simulink model "Car"  (R2023a)
settings: Solver=ode45  StartTime=0.0  StopTime=PROFILE_LENGTH  MaxStep=300.0  RelTol=1e-3
values from neighbouring files (symbols this model uses):
  AIR_DENSITY = 1.2    [Setup.m]
  C_ROLLING_RESISTANCE = .0025    (= 0.0025)    [Setup.m]
  DRAG_COEFFICIENT = 0.25    [Setup.m]
  DRIVER_DISPLAY_DRAW = 2.5    [Setup.m]
  FAN_DRAW = 4.8    [Setup.m]
  FRONTAL_AREA = 1    [Setup.m]    (also in init.m = 1.262)
  FULL_PACK_KWH = HV_PACK_VOLTAGE * HV_PACK_CAPACITY * UNIT_TO_KILO    (= 7.68)    [Setup.m]    (also in init.m)
  GRAVITY = 9.81    [Setup.m]
  HEADLIGHT_DRAW = 2    [Setup.m]
  HV_PACK_VOLTAGE = 96    [Setup.m]    (also in init.m)
  INT_CURRENTS = CURRENT_DATA_ECO(1):0.0001:CURRENT_DATA_ECO(end)    [Setup.m]
  INT_DISTANCES = DISTANCE(1):0.25:DISTANCE(end)    [Setup.m]
  INT_GRADE_ANGLE = interp1(DISTANCE, GRADE_ANGLE, INT_DISTANCES,'spline')    [Setup.m]
  INT_TORQUES_ECO = interp1(CURRENT_DATA_ECO, TORQUES_DATA_ECO, INT_CURRENTS,'spline')    [Setup.m]
  MAX_CURRENT = max(CURRENT_DATA_ECO)    [Setup.m]
  MAX_TORQUE = max(TORQUES_DATA_ECO)    [Setup.m]
  SECONDS_PER_HOUR = 3600    [Setup.m]    (also in init.m)
  START_TIME = 9*(SECONDS_PER_HOUR) + 0*(SECONDS_PER_MINUTE)    (= 32400)    [Setup.m]    (also in init.m = 0)
  STARTING_KWH = FULL_PACK_KWH * (1 - 0)    (= 7.68)    [Setup.m]    (also in init.m)
  TARGET_SPEED = 10    [Setup.m]
  TOTAL_MASS = CAR_MASS + DRIVER_MASS    (= 282.996279643)    [Setup.m]    (also in init.m)
  UNIT_TO_KILO = 1 / 1000    (= 0.001)    [Setup.m]    (also in init.m)
  WHEEL_RADIUS = WHEEL_DIAMETER_METERS / 2    (= 0.2794)    [Setup.m]
libraries: slpidlib x1
settings Model: Creator=jcpetrie  LastModifiedBy=gluo25
settings SolverCC: ZeroCrossAlgorithm=Adaptive
settings ModelReferenceCC: EnableRefExpFcnMdlSchedulingChecks=on

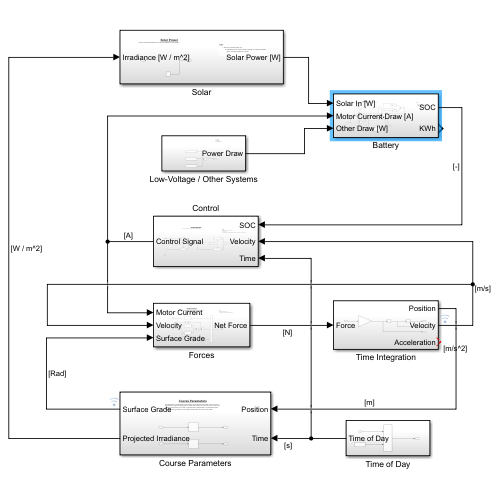
[thumbnail: Simulink's stored preview of the top-level diagram]
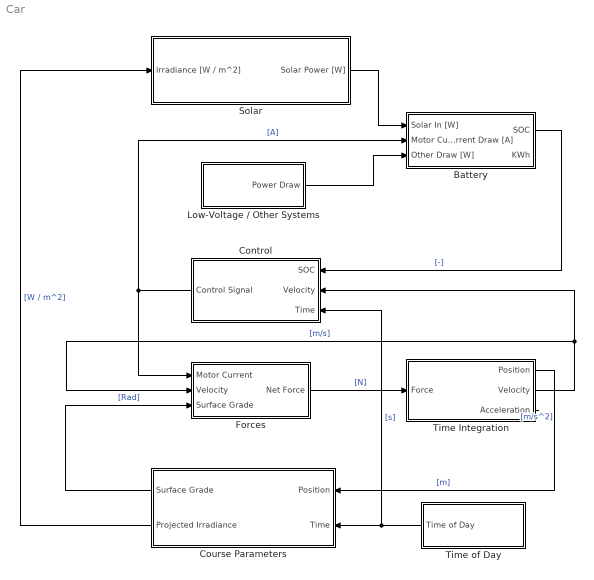
== system Car ==
  Battery : Subsystem
  Control : Subsystem
  Course Parameters : Subsystem
  Forces : Subsystem
  Low-Voltage / Other Systems : Subsystem
  Solar : Subsystem
  Time Integration : Subsystem
  Time of Day : Subsystem
  wires:
  Control/1(Control Signal) -> Battery/2(Motor Current Draw [A]), Forces/1(Motor Current)  "[A]"
  Time Integration/2(Velocity) -> Forces/2(Velocity), Control/2(Velocity)  "[m/s]"
  Forces/1(Net Force) -> Time Integration/1(Force)  "[N]"
  Time Integration/1(Position) -> Course Parameters/1(Position)  "[m]"
  Time Integration/3(Acceleration) -> ?  "[m/s^2]"
  Battery/1(SOC) -> Control/1(SOC)  "[-]"
  Course Parameters/1(Surface Grade) -> Forces/3(Surface Grade)  "[Rad]"
  Time of Day/1(Time of Day) -> Control/3(Time), Course Parameters/2(Time)  "[s]"
  Low-Voltage / Other Systems/1(Power Draw) -> Battery/3(Other Draw [W])
  Solar/1(Solar Power [W]) -> Battery/1(Solar In [W])
  Course Parameters/2(Projected Irradiance) -> Solar/1(Irradiance [W / m^2])  "[W / m^2]"

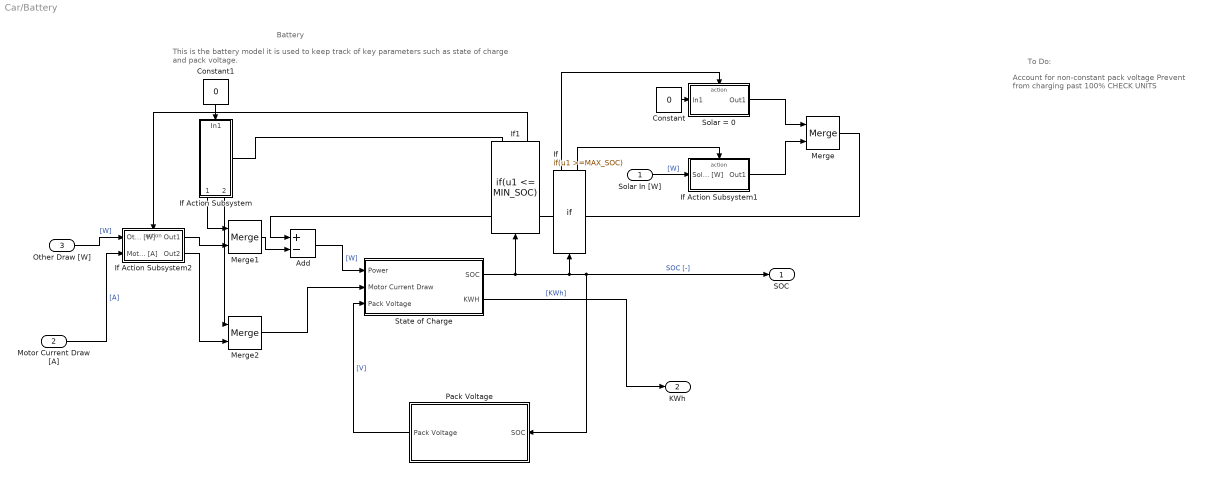
== system Car/Battery ==
  note: To Do:
  note: Battery
  note: This is the battery model it is used to keep track of key parameters such as state of charge and pack voltage.
  note: Account for non-constant pack voltage
      | Prevent from charging past 100%
      | CHECK UNITS
  Solar In [W] : Inport
  Motor Current Draw [A] : Inport  Port=2
  Other Draw [W] : Inport  Port=3
  Add : Sum  Inputs=+-
  Constant : Constant  Value=0
  Constant1 : Constant  Value=0
  If : If  IfExpression=u1 >=MAX_SOC  ZeroCross=off
  If Action Subsystem : Subsystem  TreatAsAtomicUnit=on
  If Action Subsystem1 : Subsystem  TreatAsAtomicUnit=on
  If Action Subsystem2 : Subsystem  TreatAsAtomicUnit=on
  If1 : If  IfExpression=u1 <= MIN_SOC  ZeroCross=off
  Merge : Merge
  Merge1 : Merge
  Merge2 : Merge
  Pack Voltage : Subsystem
  Solar = 0 : Subsystem  TreatAsAtomicUnit=on
  State of Charge : Subsystem
  SOC : Outport
  KWh : Outport  Port=2
  wires:
  Motor Current Draw [A]/1 -> If Action Subsystem2/2(Motor Current Draw [A])  "[A]"
  State of Charge/1(SOC) -> SOC/1, Pack Voltage/1(SOC), If/1, If1/1  "SOC [-]"
  Pack Voltage/1(Pack Voltage) -> State of Charge/3(Pack Voltage)  "[V]"
  State of Charge/2(KWH) -> KWh/1  "[KWh]"
  Solar In [W]/1 -> If Action Subsystem1/1(Solar In [W])  "[W]"
  Add/1 -> State of Charge/1("Power ")  "[W]"
  If/1 -> Solar = 0/Action
  Constant/1 -> Solar = 0/1(In1)
  If/2 -> If Action Subsystem1/Action
  Solar = 0/1(Out1) -> Merge/1
  Merge/1 -> Add/1
  Other Draw [W]/1 -> If Action Subsystem2/1(Other Draw [W])  "[W]"
  If Action Subsystem1/1(Out1) -> Merge/2
  If1/1 -> If Action Subsystem/Action
  Constant1/1 -> If Action Subsystem/1(In1)
  If1/2 -> If Action Subsystem2/Action
  If Action Subsystem2/1(Out1) -> Merge1/2
  If Action Subsystem/1(Out1) -> Merge1/1
  Merge1/1 -> Add/2
  Merge2/1 -> State of Charge/2(Motor Current Draw)
  If Action Subsystem2/2(Out2) -> Merge2/2
  If Action Subsystem/2(Out2) -> Merge2/1

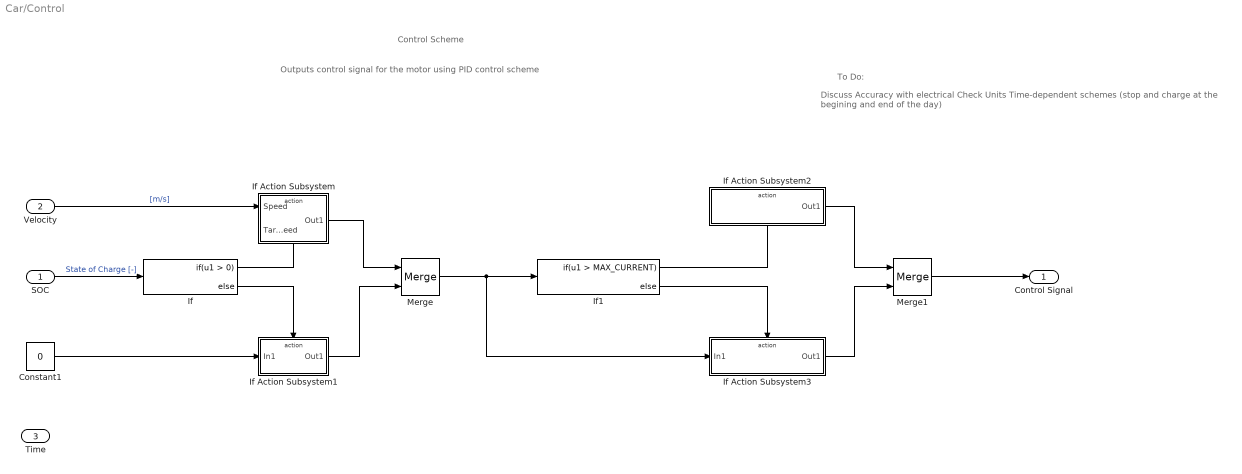
== system Car/Control ==
  note: Outputs control signal for the motor using PID control scheme
  note: To Do:
  note: Control Scheme
  note: Discuss Accuracy with electrical
      | Check Units
      | Time-dependent schemes (stop and charge at the begining and end of the day)
  SOC : Inport
  Velocity : Inport  Port=2
  Time : Inport  Port=3
  Constant1 : Constant  Value=0
  If : If  ZeroCross=off
  If Action Subsystem : Subsystem  TreatAsAtomicUnit=on
  If Action Subsystem1 : Subsystem  TreatAsAtomicUnit=on
  If Action Subsystem2 : Subsystem  TreatAsAtomicUnit=on
  If Action Subsystem3 : Subsystem  TreatAsAtomicUnit=on
  If1 : If  IfExpression=u1 > MAX_CURRENT
  Merge : Merge
  Merge1 : Merge
  Control Signal : Outport
  wires:
  Velocity/1 -> If Action Subsystem/1(Speed)  "[m/s]"
  SOC/1 -> If/1  "State of Charge [-]"
  If/1 -> If Action Subsystem/Action
  If/2 -> If Action Subsystem1/Action
  Constant1/1 -> If Action Subsystem1/1(In1)
  If Action Subsystem/1(Out1) -> Merge/1
  If Action Subsystem1/1(Out1) -> Merge/2
  Merge/1 -> If Action Subsystem3/1(In1), If1/1
  If1/1 -> If Action Subsystem2/Action
  Merge1/1 -> Control Signal/1
  If Action Subsystem2/1(Out1) -> Merge1/1
  If1/2 -> If Action Subsystem3/Action
  If Action Subsystem3/1(Out1) -> Merge1/2

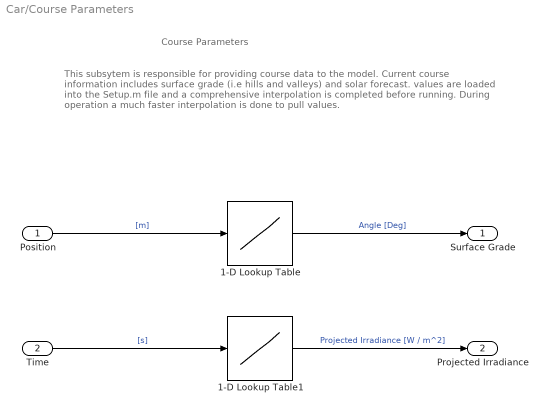
== system Car/Course Parameters ==
  note: Course Parameters
  note: This subsytem is responsible for providing course data to the model. Current course information includes surface grade (i.e hills and valleys) and solar forecast. values are loaded into the Setup.m file and a comprehensive interpolation is completed before running. During operation a much faster interpolation is done to pull values.
  Position : Inport
  Time : Inport  Port=2
  1-D Lookup Table : Lookup_n-D  NumberOfTableDimensions=1  BreakpointsForDimension1=INT_DISTANCES  Table=INT_GRADE_ANGLE  InternalRulePriority=Speed  RndMeth=Simplest
  1-D Lookup Table1 : Lookup_n-D  NumberOfTableDimensions=1  BreakpointsForDimension1=[-5:5]  Table=tanh([-5:5])  InternalRulePriority=Speed  RndMeth=Simplest
  Surface Grade : Outport
  Projected Irradiance : Outport  Port=2
  wires:
  Position/1 -> 1-D Lookup Table/1  "[m]"
  Time/1 -> 1-D Lookup Table1/1  "[s]"
  1-D Lookup Table/1 -> Surface Grade/1  "Angle [Deg]"
  1-D Lookup Table1/1 -> Projected Irradiance/1  "Projected Irradiance [W / m^2]"

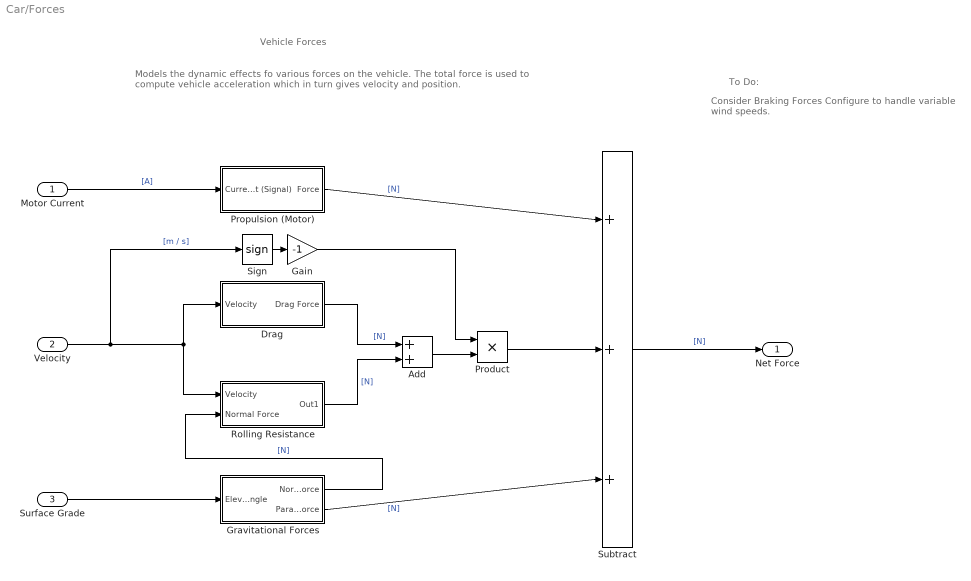
== system Car/Forces ==
  note: To Do:
  note: Vehicle Forces
  note: Models the dynamic effects fo various forces on the vehicle. The total force is used to compute vehicle acceleration which in turn gives velocity and position.
  note: Consider Braking Forces
      | Configure to handle variable wind speeds.
  Motor Current : Inport
  Velocity : Inport  Port=2
  Surface Grade : Inport  Port=3
  Add : Sum
  Drag : Subsystem
  Gain : Gain  Gain=-1
  Gravitational Forces : Subsystem
  Product : Product
  Propulsion (Motor) : Subsystem
  Rolling Resistance : Subsystem
  Sign : Signum
  Subtract : Sum  Inputs=+|+|+
  Net Force : Outport
  wires:
  Velocity/1 -> Sign/1, Drag/1(Velocity), Rolling Resistance/1(Velocity)  "[m / s]"
  Propulsion (Motor)/1(Force) -> Subtract/1  "[N]"
  Drag/1(Drag Force) -> Add/1  "[N]"
  Rolling Resistance/1(Out1) -> Add/2  "[N]"
  Subtract/1 -> Net Force/1  "[N]"
  Motor Current/1 -> Propulsion (Motor)/1(Current (Signal))  "[A]"
  Surface Grade/1 -> Gravitational Forces/1(Elevation Angle)
  Gravitational Forces/2(Parallel Force) -> Subtract/3  "[N]"
  Gravitational Forces/1(Normal Force) -> Rolling Resistance/2(Normal Force)  "[N]"
  Sign/1 -> Gain/1
  Add/1 -> Product/2
  Gain/1 -> Product/1
  Product/1 -> Subtract/2

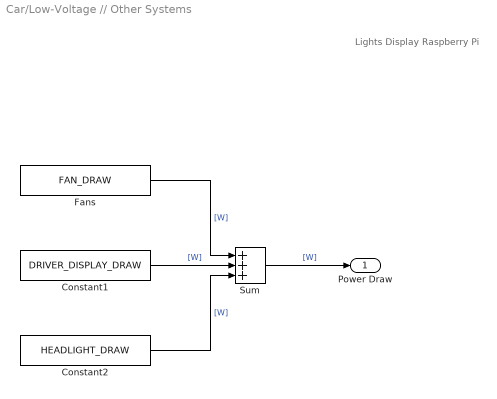
== system Car/Low-Voltage // Other Systems ==
  note: Lights
      | Display
      | Raspberry Pi
  Constant1 : Constant  Value=DRIVER_DISPLAY_DRAW
  Constant2 : Constant  Value=HEADLIGHT_DRAW
  Fans : Constant  Value=FAN_DRAW
  Sum : Sum  Inputs=+++
  Power Draw : Outport
  wires:
  Constant1/1 -> Sum/2  "[W]"
  Sum/1 -> Power Draw/1  "[W]"
  Fans/1 -> Sum/1  "[W]"
  Constant2/1 -> Sum/3  "[W]"

== system Car/Solar ==
  note: Remove constant power out
      | Replace with conversion function based on experimental data which converts irradiance to power
  note: Converts expected irradiance to solar out. Based on testing data.
  note: Solar Power
  note: To Do:
  Irradiance [W / m^2] : Inport
  Constant : Constant  Value=100
  Solar Power [W] : Outport
  wires:
  Constant/1 -> Solar Power [W]/1  "[W]"

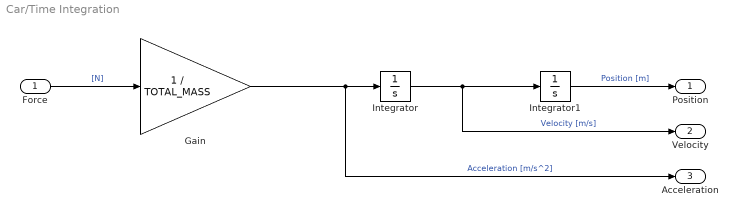
== system Car/Time Integration ==
  Force : Inport
  Gain : Gain  Gain=1 / TOTAL_MASS
  Integrator : Integrator
  Integrator1 : Integrator
  Position : Outport
  Velocity : Outport  Port=2
  Acceleration : Outport  Port=3
  wires:
  Gain/1 -> Acceleration/1, Integrator/1  "Acceleration [m/s^2]"
  Integrator/1 -> Velocity/1, Integrator1/1  "Velocity [m/s]"
  Force/1 -> Gain/1  "[N]"
  Integrator1/1 -> Position/1  "Position [m]"

== system Car/Time of Day ==
  Add : Sum
  Clock : Clock
  Constant : Constant  Value=START_TIME
  Time of Day : Outport
  wires:
  Add/1 -> Time of Day/1  "Time of Day [s]"
  Clock/1 -> Add/1  "Simulation Time [s]"
  Constant/1 -> Add/2  "Start time of day [s]"

== system Car/Battery/If Action Subsystem ==
  In1 : Inport
  Action Port : ActionPort  ActionPortLabel=if(u1 <= MIN_SOC)
  Out1 : Outport
  Out2 : Outport  Port=2
  wires:
  In1/1 -> Out2/1, Out1/1

== system Car/Battery/If Action Subsystem1 ==
  Solar In [W] : Inport
  Action Port : ActionPort  ActionPortLabel=else
  Out1 : Outport
  wires:
  Solar In [W]/1 -> Out1/1

== system Car/Battery/If Action Subsystem2 ==
  Other Draw [W] : Inport
  Motor Current Draw [A] : Inport  Port=2
  Action Port : ActionPort  ActionPortLabel=else
  Out1 : Outport
  Out2 : Outport  Port=2
  wires:
  Other Draw [W]/1 -> Out1/1
  Motor Current Draw [A]/1 -> Out2/1

== system Car/Battery/Pack Voltage ==
  note: Battery Voltage
  note: Outputs the Voltage of the battery given the state of charge
  note: To Do:
  note: Get voltage curve from battery, implment non constant behavior.
  SOC : Inport
  Constant : Constant  Value=HV_PACK_VOLTAGE
  Pack Voltage : Outport
  wires:
  SOC/1 -> ?
  Constant/1 -> Pack Voltage/1  "[V]"

== system Car/Battery/Solar = 0 ==
  In1 : Inport
  Action Port : ActionPort  ActionPortLabel=if(u1 >=MAX_SOC)
  Out1 : Outport
  wires:
  In1/1 -> Out1/1

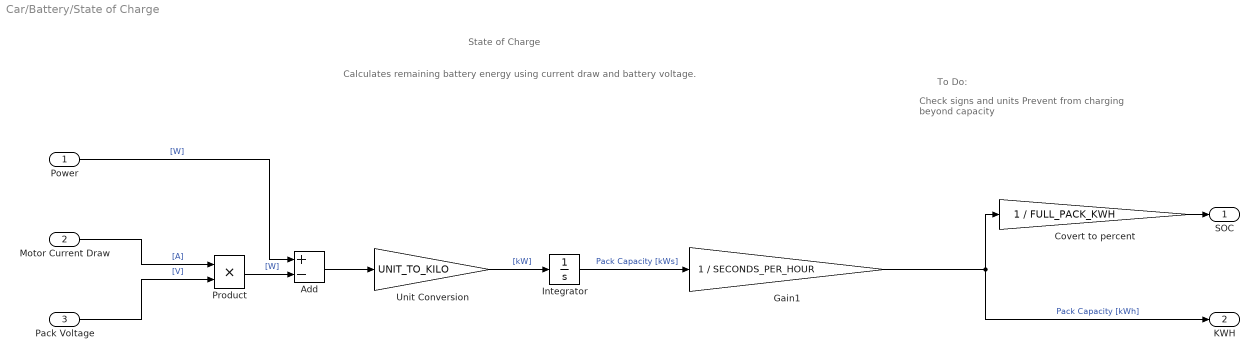
== system Car/Battery/State of Charge ==
  note: State of Charge
  note: Check signs and units
      | Prevent from charging beyond capacity
  note: To Do:
  note: Calculates remaining battery energy using current draw and battery voltage.
  "Power " : Inport
  Motor Current Draw : Inport  Port=2
  Pack Voltage : Inport  Port=3
  Add : Sum  Inputs=+-
  Covert to percent : Gain  Gain=1 / FULL_PACK_KWH
  Gain1 : Gain  Gain=1 / SECONDS_PER_HOUR
  Integrator : Integrator  InitialCondition=STARTING_KWH * SECONDS_PER_HOUR
  Product : Product  Inputs=**
  Unit Conversion : Gain  Gain=UNIT_TO_KILO
  SOC : Outport
  KWH : Outport  Port=2
  wires:
  Integrator/1 -> Gain1/1  "Pack Capacity [kWs]"
  Covert to percent/1 -> SOC/1
  Pack Voltage/1 -> Product/2  "[V]"
  Product/1 -> Add/2  "[W]"
  Unit Conversion/1 -> Integrator/1  "[kW]"
  Motor Current Draw/1 -> Product/1  "[A]"
  Gain1/1 -> KWH/1, Covert to percent/1  "Pack Capacity [kWh]"
  "Power "/1 -> Add/1  "[W]"
  Add/1 -> Unit Conversion/1

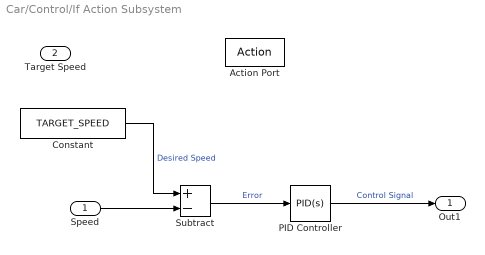
== system Car/Control/If Action Subsystem ==
  Speed : Inport
  Target Speed : Inport  Port=2
  Action Port : ActionPort  ActionPortLabel=if(u1 > 0)
  Constant : Constant  Value=TARGET_SPEED
  PID Controller : slpidlib/PID Controller  Controller=PID  Form=Parallel  TimeDomain=Continuous-time  UseExternalTs=off  SampleTime=-1  IntegratorMethod=Forward Euler  FilterMethod=Forward Euler  ControllerParametersSource=internal  P=2.5  I=0.1  UseKiTs=off  D=0  N=100  UseFilter=on  TunerSelectOption=Transfer Function Based (PID Tuner App)  InitialConditionSource=internal  InitialConditionForIntegrator=0  InitialConditionForFilter=0  DifferentiatorICPrevScaledInput=0  ExternalReset=none  TrackingMode=off  Kt=1  LimitOutput=off  SatLimitsSource=internal  UpperSaturationLimit=inf  LowerSaturationLimit=-inf  LinearizeAsGain=on  AntiWindupMode=none  Kb=1  LimitIntegrator=off  UpperIntegratorSaturationLimit=inf  LowerIntegratorSaturationLimit=-inf  POutMin=[]  POutMax=[]  IOutMin=[]  IOutMax=[]  DOutMin=[]  DOutMax=[]  NOutMin=[]  NOutMax=[]  SumOutMin=[]  SumOutMax=[]  SaturationOutMin=[]  SaturationOutMax=[]  PParamMin=[]  PParamMax=[]  IParamMin=[]  IParamMax=[]  DParamMin=[]  DParamMax=[]  NParamMin=[]  NParamMax=[]  KbParamMin=[]  KbParamMax=[]  KtParamMin=[]  KtParamMax=[]  KbOutMin=[]  KbOutMax=[]  KtOutMin=[]  KtOutMax=[]  IntegratorOutMin=[]  IntegratorOutMax=[]  FilterOutMin=[]  FilterOutMax=[]  SumI1OutMin=[]  SumI1OutMax=[]  SumI2OutMin=[]  SumI2OutMax=[]  SumI3OutMin=[]  SumI3OutMax=[]  SumI4OutMin=[]  SumI4OutMax=[]  SumDOutMin=[]  SumDOutMax=[]  DifferentiatorOutMin=[]  DifferentiatorOutMax=[]  FilterDiffOutCoefMin=[]  FilterDiffOutCoefMax=[]  ReciprocalOutMin=[]  ReciprocalOutMax=[]  SumDenOutMin=[]  SumDenOutMax=[]  SumNumOutMin=[]  SumNumOutMax=[]  DivideOutMin=[]  DivideOutMax=[]  UdiffTsProdOutMin=[]  UdiffTsProdOutMax=[]  NTsProdOutMin=[]  NTsProdOutMax=[]  UintegralTsProdOutMin=[]  UintegralTsProdOutMax=[]  UngainTsProdOutMin=[]  UngainTsProdOutMax=[]  ClampingZeroOutDataTypeStr=Inherit: Inherit via back propagation  ClampingZeroOutMin=[]  ClampingZeroOutMax=[]  FilterDenConstantOutDataTypeStr=Inherit: Inherit via back propagation  FilterDenConstantOutMin=[]  FilterDenConstantOutMax=[]  PCopyOutDataTypeStr=Inherit: Inherit via back propagation  PCopyOutMin=[]  PCopyOutMax=[]  NCopyOutDataTypeStr=Inherit: Inherit via back propagation  NCopyOutMin=[]  NCopyOutMax=[]  IntegratorContinuousStateAttributes=''  IntegratorStateMustResolveToSignalObject=off  IntegratorRTWStateStorageClass=Auto  FilterContinuousStateAttributes=''  FilterStateMustResolveToSignalObject=off  FilterRTWStateStorageClass=Auto  ParallelPVariant=InternalParameters  IdealPVariant=Disabled  IVariant=InternalParameters  DVariant=InternalParameters  IntegratorVariant=Continuous  SatVariant=Disabled  AWVariant=Passthrough  PCopyVariant=Disabled  TRVariant=Disabled  FdbkBlocksVariant=Forward  IdealPFdbkVariant=Disabled  SatFdbkVariant=Disabled  DerivativeFilterVariant=ContFilter  NVariant=InternalParameters  NCopyVariant=Disabled  FilterICVariant=InternalICsFilter  IntegratorICVariant=InternalICs  ExternalResetVariant=Disabled  TRSumVariant=Passthrough  SumFdbkVariant=Disabled  SumVariant=Sum_PID  TsampFilterVariant=InternalTs  TsampNgainVariant=Passthrough  TsampIntegralVariant=Disabled_SignalSpec  ExternalSaturationOutDataTypeStr=Inherit: Same as second input
  Subtract : Sum  Inputs=+-
  Out1 : Outport
  wires:
  Speed/1 -> Subtract/2
  PID Controller/1 -> Out1/1  "Control Signal"
  Constant/1 -> Subtract/1  "Desired Speed"
  Subtract/1 -> PID Controller/1  "Error"

== system Car/Control/If Action Subsystem1 ==
  In1 : Inport
  Action Port : ActionPort  ActionPortLabel=else
  Out1 : Outport
  wires:
  In1/1 -> Out1/1

== system Car/Control/If Action Subsystem2 ==
  Action Port : ActionPort  ActionPortLabel=if(u1 > MAX_CURRENT)
  Constant : Constant  Value=MAX_CURRENT
  Out1 : Outport
  wires:
  Constant/1 -> Out1/1

== system Car/Control/If Action Subsystem3 ==
  In1 : Inport
  Action Port : ActionPort  ActionPortLabel=else
  Out1 : Outport
  wires:
  In1/1 -> Out1/1

== system Car/Forces/Drag ==
  note: $C_d \rightarrow C_d(u)$
  note: Find the velocity dependence of the drag coefficient. Effectively we want to transform
  note: $\rho = \text{Air density} \qquad \text{(Setup.m)} \\ A = \text{Vehicle frontal area} \qquad \text{(Setup.m)} \\ C_d = \text{Vehicle drag coefficient} \qquad \text{(Calculated)} \\ u = \text{Vehicle speed} \qquad \text{(Subsystem Input)}$
  note: Where,
  note: $F_D = \frac{1}{2} \rho A C_d u^2$
  note: This computes the drag force on the vehicle due to motion using the formula
  note: To Do:
  note: Drag Force
  Velocity : Inport
  0.5 rho A : Gain  Gain=0.5 * AIR_DENSITY * FRONTAL_AREA
  Drag Coefficient : Gain  Gain=DRAG_COEFFICIENT
  Square : Math  Operator=square
  Drag Force : Outport
  wires:
  Velocity/1 -> Square/1  "[m / s]"
  Square/1 -> 0.5 rho A/1  "[m^2/s^2]"
  0.5 rho A/1 -> Drag Coefficient/1  "[N]"
  Drag Coefficient/1 -> Drag Force/1  "[N]"

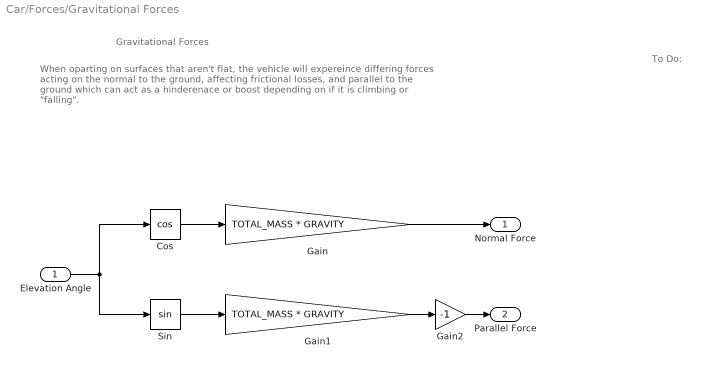
== system Car/Forces/Gravitational Forces ==
  note: To Do:
  note: Gravitational Forces
  note: When oparting on surfaces that aren't flat, the vehicle will expereince differing forces acting on the normal to the ground, affecting frictional losses, and parallel to the ground which can act as a hinderenace or boost depending on if it is climbing or "falling".
  Elevation Angle : Inport
  Cos : Trigonometry  Operator=cos
  Gain : Gain  Gain=TOTAL_MASS * GRAVITY
  Gain1 : Gain  Gain=TOTAL_MASS * GRAVITY
  Gain2 : Gain  Gain=-1
  Sin : Trigonometry
  Normal Force : Outport
  Parallel Force : Outport  Port=2
  wires:
  Elevation Angle/1 -> Sin/1, Cos/1
  Cos/1 -> Gain/1
  Gain/1 -> Normal Force/1
  Sin/1 -> Gain1/1
  Gain1/1 -> Gain2/1
  Gain2/1 -> Parallel Force/1

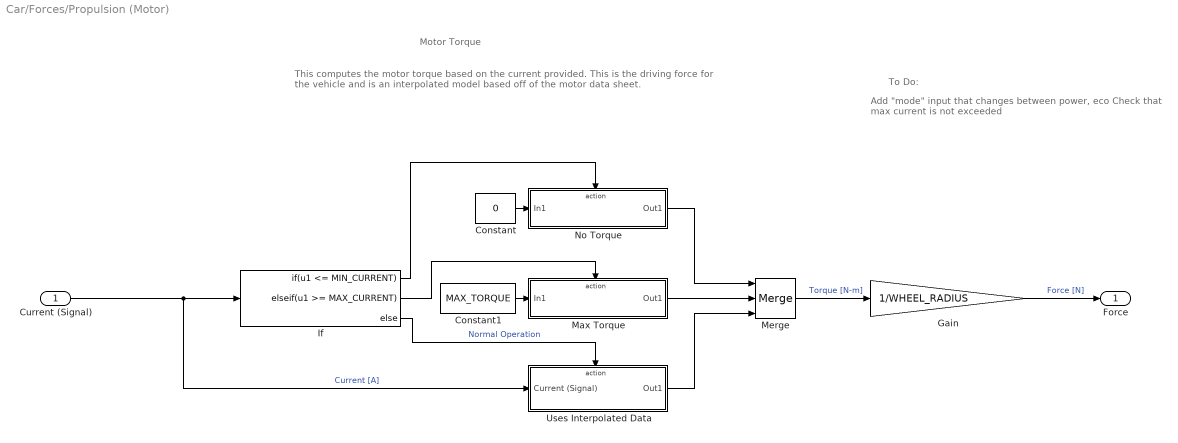
== system Car/Forces/Propulsion (Motor) ==
  note: Add "mode" input that changes between power, eco
      | Check that max current is not exceeded
  note: Motor Torque
  note: To Do:
  note: This computes the motor torque based on the current provided. This is the driving force for the vehicle and is an interpolated model based off of the motor data sheet.
  Current (Signal) : Inport
  Constant : Constant  Value=0
  Constant1 : Constant  Value=MAX_TORQUE
  Gain : Gain  Gain=1/WHEEL_RADIUS
  If : If  IfExpression=u1 <= MIN_CURRENT  ElseIfExpressions=u1 >= MAX_CURRENT
  Max Torque : Subsystem  TreatAsAtomicUnit=on
  Merge : Merge  Inputs=3
  No Torque : Subsystem  TreatAsAtomicUnit=on
  Uses Interpolated Data : Subsystem  TreatAsAtomicUnit=on
  Force : Outport
  wires:
  Current (Signal)/1 -> Uses Interpolated Data/1(Current (Signal)), If/1  "Current [A]"
  Constant/1 -> No Torque/1(In1)
  If/1 -> No Torque/Action
  If/2 -> Max Torque/Action
  Uses Interpolated Data/1(Out1) -> Merge/3
  No Torque/1(Out1) -> Merge/1
  Merge/1 -> Gain/1  "Torque [N-m]"
  If/3 -> Uses Interpolated Data/Action  "Normal Operation"
  Constant1/1 -> Max Torque/1(In1)
  Max Torque/1(Out1) -> Merge/2
  Gain/1 -> Force/1  "Force [N]"

== system Car/Forces/Rolling Resistance ==
  note: This computes the rolling resitance on the vehicle due to motion using the formula
  note: To Do:
  note: $C_{RR} = \text{Coefficient of Rolling Resistance \quad (Reddit)} \\ N = \text{Normal Force \quad (Weight)}$
  note: Where,
  note: Find the velocity dependence of the rolling resistance coefficient. Effectively we want to transform
      | Account for elevation changes
  note: Rolling Resistance
  note: $F_{RR} = C_{RR} N$
  Velocity : Inport
  Normal Force : Inport  Port=2
  Constant : Constant  Value=C_ROLLING_RESISTANCE
  Product : Product
  Out1 : Outport
  wires:
  Velocity/1 -> ?
  Constant/1 -> Product/1  "[-]"
  Product/1 -> Out1/1  "[N]"
  Normal Force/1 -> Product/2  "[N]"

== system Car/Forces/Propulsion (Motor)/Max Torque ==
  In1 : Inport
  Action Port : ActionPort  ActionPortLabel=elseif(u1 >= MAX_CURRENT)
  Out1 : Outport
  wires:
  In1/1 -> Out1/1

== system Car/Forces/Propulsion (Motor)/No Torque ==
  In1 : Inport
  Action Port : ActionPort  ActionPortLabel=if(u1 <= MIN_CURRENT)
  Out1 : Outport
  wires:
  In1/1 -> Out1/1

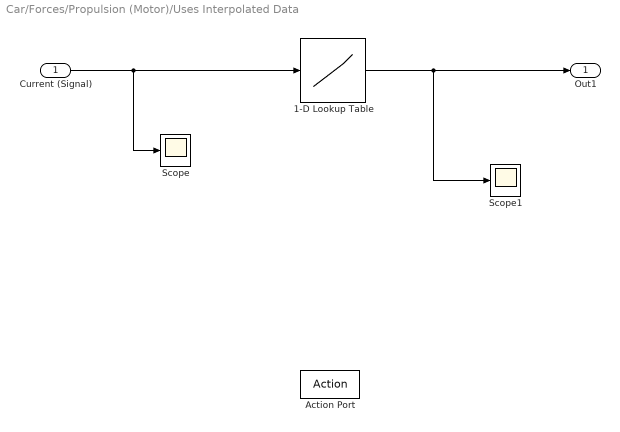
== system Car/Forces/Propulsion (Motor)/Uses Interpolated Data ==
  Current (Signal) : Inport
  Action Port : ActionPort  ActionPortLabel=else
  1-D Lookup Table : Lookup_n-D  NumberOfTableDimensions=1  LookupTableObject=''  BreakpointsForDimension1=INT_CURRENTS  BreakpointsForDimension1FirstPoint=10  BreakpointsForDimension2FirstPoint=10  BreakpointsForDimension1Spacing=12  BreakpointsForDimension2Spacing=12  Table=INT_TORQUES_ECO  DiagnosticForOutOfRangeInput=Warning  InternalRulePriority=Speed  RndMeth=Simplest
  Scope : Scope
  Scope1 : Scope
  Out1 : Outport
  wires:
  Current (Signal)/1 -> Scope/1, 1-D Lookup Table/1
  1-D Lookup Table/1 -> Scope1/1, Out1/1
